simulink model "a1_climbing_new_swing"  (R2022b)
settings: Solver=ode15s  StartTime=0.0  StopTime=10  RelTol=1e-3
values from neighbouring files (symbols this model uses):
  m = 12    [MPC_Controller.m]    (also in QP_Controller.m; TASK1_rotating_mpc.m; TASK1_walking_backward_mpc.m; TASK1_walking_forward_mpc.m)
  N = 10    [MPC_Controller.m]
undefined symbols (not defined in the file or in its folder): climbing_mpc, square_trajectory_t_end, X, Y, Z
libraries: sm_lib x207, nesl_utility x134, simulink x1
(part 6 of 6)

== system a1_climbing_new_swing/Stand Controller/Subsystem9 ==
  angle : Inport
  velocity : Inport  Port=2
  Add : Sum
  Constant1 : Constant  Value=-0.5
  Constant2 : Constant  Value=-5
  Constant3 : Constant  Value=0
  Product : Product
  Product1 : Product
  Saturation : Saturate  UpperLimit=33.5  LowerLimit=-33.5
  Subtract : Sum  Inputs=+-
  Torque : Outport
  wires:
  angle/1 -> Subtract/1
  Constant2/1 -> Product/2
  Subtract/1 -> Product/1
  Constant1/1 -> Product1/2
  velocity/1 -> Product1/1
  Product1/1 -> Add/2
  Product/1 -> Add/1
  Constant3/1 -> Subtract/2
  Add/1 -> Saturation/1
  Saturation/1 -> Torque/1

== system a1_climbing_new_swing/Walk Controller/Convert Forces to Torque1 ==
  F : Inport
  RR_Ang_Vec : Inport  Port=2
  RL_Ang_Vec : Inport  Port=3
  FL_Ang_Vec : Inport  Port=4
  FR_Ang_Vec : Inport  Port=5
  Force to Torque : MATLAB Function  TreatAsAtomicUnit=on
  Tau_FL : Outport
  Tau_RL : Outport  Port=2
  Tau_FR : Outport  Port=3
  Tau_RR : Outport  Port=4
  wires:
  F/1 -> Force to Torque/1(F)
  Force to Torque/1(Tau_RR) -> Tau_RR/1
  Force to Torque/2(Tau_FR) -> Tau_FR/1
  Force to Torque/3(Tau_FL) -> Tau_FL/1
  Force to Torque/4(Tau_RL) -> Tau_RL/1
  RR_Ang_Vec/1 -> Force to Torque/2(RR_ang_vec)
  RL_Ang_Vec/1 -> Force to Torque/3(RL_ang_vec)
  FL_Ang_Vec/1 -> Force to Torque/4(FL_ang_vec)
  FR_Ang_Vec/1 -> Force to Torque/5(FR_ang_vec)

== system a1_climbing_new_swing/Walk Controller/Rigid Body Controller ==
  FL Pos : Inport
  RL Pos : Inport  Port=2
  FR Pos : Inport  Port=3
  RR Pos : Inport  Port=4
  COM_pos : Inport  Port=5
  COM_vel : Inport  Port=6
  COM_ang_vel : Inport  Port=7
  Rot : Inport  Port=8
  v_desired : Inport  Port=9
  T_stance : Inport  Port=10
  Clock : Clock
  Interpreted MATLAB Function : MATLABFcn  MATLABFcn=climbing_mpc(u)  OutputDimensions=12  Output1D=off
  Memory : Memory
  Mux : Mux  Inputs=11
  Rotation Matrix to Eul : MATLAB Function  TreatAsAtomicUnit=on
  Scope : Scope  NumInputPorts=5
  Selector : Selector  InputPortWidth=12  IndexOptions=Index vector (dialog)  Indices=[1 3]  OutputSizes=1
  Zero-Order Hold : ZeroOrderHold  SampleTime=.05
  u : Outport
  wires:
  COM_pos/1 -> Mux/1
  COM_vel/1 -> Mux/2
  COM_ang_vel/1 -> Mux/4
  FL Pos/1 -> Mux/5
  RL Pos/1 -> Mux/6
  FR Pos/1 -> Mux/7
  RR Pos/1 -> Mux/8
  Rot/1 -> Rotation Matrix to Eul/1(u)
  Rotation Matrix to Eul/1(y) -> Mux/3
  Interpreted MATLAB Function/1 -> Memory/1
  Memory/1 -> Selector/1, u/1
  Mux/1 -> Zero-Order Hold/1
  Zero-Order Hold/1 -> Interpreted MATLAB Function/1
  Clock/1 -> Mux/9
  Selector/1 -> Scope/1
  v_desired/1 -> Mux/10
  T_stance/1 -> Mux/11

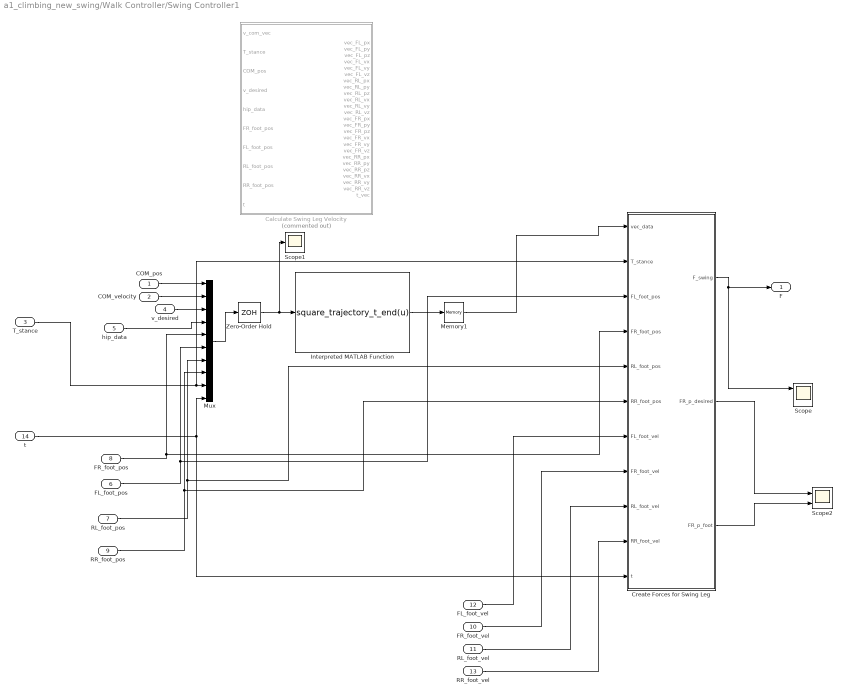
== system a1_climbing_new_swing/Walk Controller/Swing Controller1 ==
  COM_pos : Inport
  COM_velocity : Inport  Port=2
  T_stance : Inport  Port=3
  v_desired : Inport  Port=4
  hip_data : Inport  Port=5
  FL_foot_pos : Inport  Port=6
  RL_foot_pos : Inport  Port=7
  FR_foot_pos : Inport  Port=8
  RR_foot_pos : Inport  Port=9
  FR_foot_vel : Inport  Port=10
  RL_foot_vel : Inport  Port=11
  FL_foot_vel : Inport  Port=12
  RR_foot_vel : Inport  Port=13
  t : Inport  Port=14
  Calculate Swing Leg Velocity : MATLAB Function  Commented=on  TreatAsAtomicUnit=on
  Create Forces for Swing Leg : MATLAB Function  TreatAsAtomicUnit=on
  Interpreted MATLAB Function : MATLABFcn  MATLABFcn=square_trajectory_t_end(u)  OutputDimensions=1025  Output1D=off
  Memory1 : Memory
  Mux : Mux  Inputs=10
  Scope : Scope  NumInputPorts=3
  Scope1 : Scope
  Scope2 : Scope  NumInputPorts=2
  Zero-Order Hold : ZeroOrderHold  SampleTime=.2
  F : Outport
  wires:
  Create Forces for Swing Leg/1(F_swing) -> Scope/1, F/1
  t/1 -> Mux/10, Create Forces for Swing Leg/11(t)
  FR_foot_pos/1 -> Mux/5, Create Forces for Swing Leg/4(FR_foot_pos)
  RL_foot_pos/1 -> Mux/7, Create Forces for Swing Leg/5(RL_foot_pos)
  RR_foot_pos/1 -> Create Forces for Swing Leg/6(RR_foot_pos), Mux/8
  FL_foot_vel/1 -> Create Forces for Swing Leg/7(FL_foot_vel)
  FR_foot_vel/1 -> Create Forces for Swing Leg/8(FR_foot_vel)
  RL_foot_vel/1 -> Create Forces for Swing Leg/9(RL_foot_vel)
  RR_foot_vel/1 -> Create Forces for Swing Leg/10(RR_foot_vel)
  Create Forces for Swing Leg/2(FR_p_desired) -> Scope2/1
  Create Forces for Swing Leg/3(FR_p_foot) -> Scope2/2
  FL_foot_pos/1 -> Mux/6, Create Forces for Swing Leg/3(FL_foot_pos)
  Interpreted MATLAB Function/1 -> Memory1/1
  Zero-Order Hold/1 -> Scope1/1, Interpreted MATLAB Function/1
  COM_pos/1 -> Mux/1
  COM_velocity/1 -> Mux/2
  v_desired/1 -> Mux/3
  hip_data/1 -> Mux/4
  T_stance/1 -> Create Forces for Swing Leg/2(T_stance), Mux/9
  Mux/1 -> Zero-Order Hold/1
  Memory1/1 -> Create Forces for Swing Leg/1(vec_data)

== matlab function a1_climbing_new_swing/Rear Left Leg/Separate Torques ==
  data: torque_vector input; hip_torque output; thigh_torque output; calf_torque output
function [hip_torque, thigh_torque, calf_torque] = fcn(torque_vector)

hip_torque = torque_vector(1);
thigh_torque = torque_vector(2);
calf_torque = torque_vector(3);

== matlab function a1_climbing_new_swing/Front Right Leg/Separate Torques ==
  data: torque_vector input; hip_torque output; thigh_torque output; calf_torque output
function [hip_torque, thigh_torque, calf_torque] = fcn(torque_vector)

hip_torque = torque_vector(1);
thigh_torque = torque_vector(2);
calf_torque = torque_vector(3);

== matlab function a1_climbing_new_swing/Rear Right Leg/Separate Torques ==
  data: torque_vector input; hip_torque output; thigh_torque output; calf_torque output
function [hip_torque, thigh_torque, calf_torque] = fcn(torque_vector)

hip_torque = torque_vector(1);
thigh_torque = torque_vector(2);
calf_torque = torque_vector(3);

== matlab function a1_climbing_new_swing/Front Left Leg/Separate Torques ==
  data: torque_vector input; hip_torque output; thigh_torque output; calf_torque output
function [hip_torque, thigh_torque, calf_torque] = fcn(torque_vector)

hip_torque = torque_vector(1);
thigh_torque = torque_vector(2);
calf_torque = torque_vector(3);

== matlab function a1_climbing_new_swing/Stand Controller/MATLAB Function ==
  data: angle_vector input; hip_angle output; thigh_angle output; calf_angle output
function [hip_angle, thigh_angle, calf_angle] = fcn(angle_vector)

hip_angle = angle_vector(1);
thigh_angle = angle_vector(2);
calf_angle = angle_vector(3);

== matlab function a1_climbing_new_swing/Stand Controller/MATLAB Function1 ==
  data: velocity_vector input; hip_velocity output; thigh_velocity output; calf_velocity output
function [hip_velocity, thigh_velocity, calf_velocity] = fcn(velocity_vector)

hip_velocity = velocity_vector(1);
thigh_velocity = velocity_vector(2);
calf_velocity = velocity_vector(3);

== matlab function a1_climbing_new_swing/Stand Controller/MATLAB Function2 ==
  data: angle_vector input; hip_angle output; thigh_angle output; calf_angle output
function [hip_angle, thigh_angle, calf_angle] = fcn(angle_vector)

hip_angle = angle_vector(1);
thigh_angle = angle_vector(2);
calf_angle = angle_vector(3);

== matlab function a1_climbing_new_swing/Stand Controller/MATLAB Function3 ==
  data: velocity_vector input; hip_velocity output; thigh_velocity output; calf_velocity output
function [hip_velocity, thigh_velocity, calf_velocity] = fcn(velocity_vector)

hip_velocity = velocity_vector(1);
thigh_velocity = velocity_vector(2);
calf_velocity = velocity_vector(3);

== matlab function a1_climbing_new_swing/Stand Controller/MATLAB Function4 ==
  data: angle_vector input; hip_angle output; thigh_angle output; calf_angle output
function [hip_angle, thigh_angle, calf_angle] = fcn(angle_vector)

hip_angle = angle_vector(1);
thigh_angle = angle_vector(2);
calf_angle = angle_vector(3);

== matlab function a1_climbing_new_swing/Stand Controller/MATLAB Function5 ==
  data: velocity_vector input; hip_velocity output; thigh_velocity output; calf_velocity output
function [hip_velocity, thigh_velocity, calf_velocity] = fcn(velocity_vector)

hip_velocity = velocity_vector(1);
thigh_velocity = velocity_vector(2);
calf_velocity = velocity_vector(3);

== matlab function a1_climbing_new_swing/Stand Controller/MATLAB Function6 ==
  data: angle_vector input; hip_angle output; thigh_angle output; calf_angle output
function [hip_angle, thigh_angle, calf_angle] = fcn(angle_vector)

hip_angle = angle_vector(1);
thigh_angle = angle_vector(2);
calf_angle = angle_vector(3);

== matlab function a1_climbing_new_swing/Stand Controller/MATLAB Function7 ==
  data: velocity_vector input; hip_velocity output; thigh_velocity output; calf_velocity output
function [hip_velocity, thigh_velocity, calf_velocity] = fcn(velocity_vector)

hip_velocity = velocity_vector(1);
thigh_velocity = velocity_vector(2);
calf_velocity = velocity_vector(3);

== matlab function a1_climbing_new_swing/Walk Controller/Combine Forces ==
  data: t input; T_stance input; F output; rigid_body_forces input; swing_forces input; Contact input; Stair_Cont input
function F = fcn(t, T_stance, rigid_body_forces, swing_forces, Contact, Stair_Cont)
%#codegen
intervals = 0:T_stance:10;

interval_idx = discretize(t, intervals);
Stair1_Cont = Stair_Cont(1:4); Stair2_Cont = Stair_Cont(5:8); 


if Contact(1) == 0 && Stair1_Cont(1) == 0 && Stair2_Cont(1) == 0
    rigid_body_forces(1) = 0; 
end
if Contact(2) == 0 && Stair1_Cont(2) == 0 && Stair2_Cont(2) == 0 
    rigid_body_forces(4) = 0; 
end
if Contact(3) == 0 && Stair1_Cont(3) == 0 && Stair2_Cont(3) == 0 
    rigid_body_forces(7) = 0; 
end
if Contact(4) == 0 && Stair1_Cont(4) == 0 && Stair2_Cont(4) == 0 
    rigid_body_forces(10) = 0; 
end

if mod(interval_idx(1), 2) == 0
    F = [rigid_body_forces(1:3); -swing_forces(4:6); -swing_forces(7:9); rigid_body_forces(10:12)];
else
    F = [-swing_forces(1:3); rigid_body_forces(4:6); rigid_body_forces(7:9); -swing_forces(10:12)];
end

== matlab function a1_climbing_new_swing/Walk Controller/Rigid Body Controller/Rotation Matrix to Eul ==
  data: u input; y output
function y = fcn(u)
y = rotm2eul(u);

== matlab function a1_climbing_new_swing/Walk Controller/Swing Controller1/Calculate Swing Leg Velocity ==
  settings: updateMethod=CONTINUOUS
  data: vec_FL_px output size=41; vec_FL_py output size=41 [1..1000]; v_com_vec input; vec_FL_pz output size=41 [1..1000]; T_stance input; COM_pos input; v_desired input; hip_data input; FR_foot_pos input; FL_foot_pos input; RL_foot_pos input; vec_FL_vx output size=41; vec_FL_vy output size=41; vec_FL_vz output size=41; vec_RL_px output size=41; vec_RL_py output size=41; vec_RL_pz output size=41; vec_RL_vx output size=41; vec_RL_vy output size=41; vec_RL_vz output size=41; vec_FR_px output size=41; vec_FR_py output size=41; vec_FR_pz output size=41; vec_FR_vx output size=41; vec_FR_vy output size=41; vec_FR_vz output size=41; vec_RR_px output size=41; vec_RR_py output size=41; vec_RR_pz output size=41; vec_RR_vx output size=41; vec_RR_vy output size=41; vec_RR_vz output size=41; t_vec output size=41; RR_foot_pos input; t input
function [vec_FL_px,vec_FL_py,vec_FL_pz,vec_FL_vx,vec_FL_vy,vec_FL_vz,vec_RL_px,vec_RL_py,vec_RL_pz,vec_RL_vx,vec_RL_vy,vec_RL_vz,vec_FR_px,vec_FR_py,vec_FR_pz,vec_FR_vx,vec_FR_vy,vec_FR_vz,vec_RR_px,vec_RR_py,vec_RR_pz,vec_RR_vx,vec_RR_vy,vec_RR_vz,t_vec] = fcn(v_com_vec,T_stance,COM_pos,v_desired,hip_data,FR_foot_pos,FL_foot_pos,RL_foot_pos,RR_foot_pos,t)

z_height = 0.12; 

FL_hip_pos = hip_data(1:3);
FR_hip_pos = hip_data(4:6);
RL_hip_pos = hip_data(7:9);
RR_hip_pos = hip_data(10:12);
y_offset = 0.09; 

% Find K_step - this value can be tuned with z_com_desired
z_com_desired = 0.3;
t_delta = 0.005; 
g = 9.81;
K_step = sqrt(z_com_desired/g);

%% FL
% Find P_foot_desired - FL
FL_hip_pos(3) = 0;
FL_p_foot_desired_end = FL_hip_pos+(T_stance/2)*v_desired+K_step*(v_com_vec-v_desired);
FL_p_foot_desired_end(2) = FL_p_foot_desired_end(2)+y_offset;

if FL_p_foot_desired_end(1) > 0.4
    FL_p_foot_desired_end(3) = 0.1;
    half_step = (FL_p_foot_desired_end - FL_foot_pos)/2+[0;0;z_height];
elseif FL_p_foot_desired_end(1) > 0.6
    FL_p_foot_desired_end(3) = 0.2;
    half_step = (FL_p_foot_desired_end - FL_foot_pos)/2+[0;0;z_height];
else
   FL_p_foot_desired_end(3) = 0;
   half_step = (FL_p_foot_desired_end - FL_foot_pos)/2+[0;0;z_height];
end

% Create Velocity  
half_step_time = T_stance/2;
v = half_step/half_step_time;

% Create Trajectory Vectors
i = 1; 
vec_leng = 0:t_delta:T_stance;

vec_FL_px = zeros(1,length(vec_leng));
vec_FL_py = zeros(1,length(vec_leng));
vec_FL_pz = zeros(1,length(vec_leng));
vec_FL_vx = zeros(1,length(vec_leng));
vec_FL_vy = zeros(1,length(vec_leng));
vec_FL_vz = zeros(1,length(vec_leng));
t_vec = zeros(1,length(vec_leng));

for t = 0:t_delta:T_stance
    vec_FL_px(i) = v(1)*t;
    vec_FL_py(i) = v(2)*t;
    vec_FL_pz(i) = v(3)*t;
    vec_FL_vx(i) = v(1);
    vec_FL_vy(i) = v(2);
    vec_FL_vz(i) = v(3);
    t_vec(i) = t;
    if vec_FL_pz(i) > z_height
        vec_FL_pz(i) = z_height-v(3)*(t-T_stance/2);
        vec_FL_vz(i) = -v(3);
    end
    i = i+1; 
end

%% FR
% Find P_foot_desired - FR
FR_hip_pos(3) = 0;
FR_p_foot_desired_end = FR_hip_pos+(T_stance/2)*v_desired+K_step*(v_com_vec-v_desired);
FR_p_foot_desired_end(2) = FR_p_foot_desired_end(2)-y_offset;

if FR_p_foot_desired_end(1) > 0.4
    FR_p_foot_desired_end(3) = 0.1;
    half_step = (FR_p_foot_desired_end - FR_foot_pos)/2+[0;0;z_height];
elseif FR_p_foot_desired_end(1) > 0.6
    FR_p_foot_desired_end(3) = 0.2;
    half_step = (FR_p_foot_desired_end - FR_foot_pos)/2+[0;0;z_height];
else
   FR_p_foot_desired_end(3) = 0;
   half_step = (FR_p_foot_desired_end - FR_foot_pos)/2+[0;0;z_height];
end


% Create Trajectory 
half_step_time = T_stance/2;
v = half_step/half_step_time;


vec_FR_px = zeros(1,length(vec_leng));
vec_FR_py = zeros(1,length(vec_leng));
vec_FR_pz = zeros(1,length(vec_leng));
vec_FR_vx = zeros(1,length(vec_leng));
vec_FR_vy = zeros(1,length(vec_leng));
vec_FR_vz = zeros(1,length(vec_leng));

i = 1; 
for t = 0:t_delta:T_stance
    vec_FR_px(i) = v(1)*t;
    vec_FR_py(i) = v(2)*t;
    vec_FR_pz(i) = v(3)*t;
    vec_FR_vx(i) = v(1);
    vec_FR_vy(i) = v(2);
    vec_FR_vz(i) = v(3);
    if vec_FR_pz(i) > z_height
        vec_FR_pz(i) = z_height-v(3)*(t-T_stance/2);
        vec_FR_vz(i) = -v(3);
    end
    i = i+1; 
end

%% RL
% Find P_foot_desired - RL
RL_hip_pos(3) = 0;
RL_p_foot_desired_end = RL_hip_pos+(T_stance/2)*v_desired+K_step*(v_com_vec-v_desired);
RL_p_foot_desired_end(2) = RL_p_foot_desired_end(2)+y_offset;

if RL_p_foot_desired_end(1) > 0.4
    RL_p_foot_desired_end(3) = 0.1;
    half_step = (RL_p_foot_desired_end - RL_foot_pos)/2+[0;0;z_height];
elseif RL_p_foot_desired_end(1) > 0.6
    RL_p_foot_desired_end(3) = 0.2;
    half_step = (RL_p_foot_desired_end - RL_foot_pos)/2+[0;0;z_height];
else
   RL_p_foot_desired_end(3) = 0;
   half_step = (RL_p_foot_desired_end - RL_foot_pos)/2+[0;0;z_height];
end

% Create Trajectory 
half_step_time = T_stance/2;
v = half_step/half_step_time;


vec_RL_px = zeros(1,length(vec_leng));
vec_RL_py = zeros(1,length(vec_leng));
vec_RL_pz = zeros(1,length(vec_leng));
vec_RL_vx = zeros(1,length(vec_leng));
vec_RL_vy = zeros(1,length(vec_leng));
vec_RL_vz = zeros(1,length(vec_leng));
i = 1; 
for t = 0:t_delta:T_stance
    vec_RL_px(i) = v(1)*t;
    vec_RL_py(i) = v(2)*t;
    vec_RL_pz(i) = v(3)*t;
    vec_RL_vx(i) = v(1);
    vec_RL_vy(i) = v(2);
    vec_RL_vz(i) = v(3);
    if vec_RL_pz(i) > z_height
        vec_RL_pz(i) = z_height-v(3)*(t-T_stance/2);
        vec_RL_vz(i) = -v(3);
    end
    i = i+1; 
end


%% RR
% Find P_foot_desired - RR
RR_hip_pos(3) = 0;
RR_p_foot_desired_end = RR_hip_pos+(T_stance/2)*v_desired+K_step*(v_com_vec-v_desired);
RR_p_foot_desired_end(2) = RR_p_foot_desired_end(2)-y_offset;

% Create Trajectory 
if RR_p_foot_desired_end(1) > 0.4
    RR_p_foot_desired_end(3) = 0.1;
    half_step = (RR_p_foot_desired_end - RR_foot_pos)/2+[0;0;z_height];
elseif RR_p_foot_desired_end(1) > 0.6
    RR_p_foot_desired_end(3) = 0.2;
    half_step = (RR_p_foot_desired_end - RR_foot_pos)/2+[0;0;z_height];
else
   RR_p_foot_desired_end(3) = 0;
   half_step = (RR_p_foot_desired_end - RR_foot_pos)/2+[0;0;z_height];
end

half_step_time = T_stance/2;
v = half_step/half_step_time;


vec_RR_px = zeros(1,length(vec_leng));
vec_RR_py = zeros(1,length(vec_leng));
vec_RR_pz = zeros(1,length(vec_leng));
vec_RR_vx = zeros(1,length(vec_leng));
vec_RR_vy = zeros(1,length(vec_leng));
vec_RR_vz = zeros(1,length(vec_leng));
i = 1; 
for t = 0:t_delta:T_stance
    vec_RR_px(i) = v(1)*t;
    vec_RR_py(i) = v(2)*t;
    vec_RR_pz(i) = v(3)*t;
    vec_RR_vx(i) = v(1);
    vec_RR_vy(i) = v(2);
    vec_RR_vz(i) = v(3);
    if vec_FR_pz(i) > z_height
        vec_RR_pz(i) = z_height-v(3)*(t-T_stance/2);
        vec_RR_vz(i) = -v(3);
    end
    i = i+1; 
end

== matlab function a1_climbing_new_swing/Walk Controller/Swing Controller1/Create Forces for Swing Leg ==
  data: vec_data input size=[1025 1] [1..1000]; F_swing output; T_stance input; FL_foot_pos input; FR_foot_pos input; RL_foot_pos input; RR_foot_pos input; FL_foot_vel input; FR_foot_vel input; RL_foot_vel input; RR_foot_vel input; t input; FR_p_desired output; FR_p_foot output
function [F_swing,FR_p_desired,FR_p_foot]  = fcn(vec_data,T_stance,FL_foot_pos,FR_foot_pos,RL_foot_pos,RR_foot_pos,FL_foot_vel,FR_foot_vel,RL_foot_vel,RR_foot_vel,t)

% These are the desired velocity values calculated from the previous block
% These are the desired velocity for each foot position through the swing
vec_FL = vec_data(1:246);
vec_FL_px = vec_FL(1:41);
vec_FL_py = vec_FL(42:82);
vec_FL_pz = vec_FL(83:123);
vec_FL_vx = vec_FL(124:164);
vec_FL_vy = vec_FL(165:205);
vec_FL_vz = vec_FL(206:246);

vec_RL = vec_data(247:492);
vec_RL_px = vec_RL(1:41);
vec_RL_py = vec_RL(42:82);
vec_RL_pz = vec_RL(83:123);
vec_RL_vx = vec_RL(124:164);
vec_RL_vy = vec_RL(165:205);
vec_RL_vz = vec_RL(206:246);

vec_FR = vec_data(493:738);
vec_FR_px = vec_FR(1:41);
vec_FR_py = vec_FR(42:82);
vec_FR_pz = vec_FR(83:123);
vec_FR_vx = vec_FR(124:164);
vec_FR_vy = vec_FR(165:205);
vec_FR_vz = vec_FR(206:246);

vec_RR = vec_data(739:984);
vec_RR_px = vec_RR(1:41);
vec_RR_py = vec_RR(42:82);
vec_RR_pz = vec_RR(83:123);
vec_RR_vx = vec_RR(124:164);
vec_RR_vy = vec_RR(165:205);
vec_RR_vz = vec_RR(206:246);

t_vec = vec_data(985:1025);


steps = 0:T_stance:10;
step_index = discretize(t,steps);
delta_t = t-steps(step_index);

[dt index] = min(abs(t_vec-delta_t));


FL_v_desired = [vec_FL_vx(index);vec_FL_vy(index);vec_FL_vz(index)];
FR_v_desired = [vec_FR_vx(index);vec_FR_vy(index);vec_FR_vz(index)];
RL_v_desired = [vec_RL_vx(index);vec_RL_vy(index);vec_RL_vz(index)];
RR_v_desired = [vec_RR_vx(index);vec_RR_vy(index);vec_RR_vz(index)];

FL_p_desired = [vec_FL_px(index);vec_FL_py(index);vec_FL_pz(index)];
FR_p_desired = [vec_FR_px(index);vec_FR_py(index);vec_FR_pz(index)];
RL_p_desired = [vec_RL_px(index);vec_RL_py(index);vec_RL_pz(index)];
RR_p_desired = [vec_RR_px(index);vec_RR_py(index);vec_RR_pz(index)];


% These are the actual current foot position and velocity - these update
% continously
FL_p_foot = FL_foot_pos(1:3);
FL_v_foot = FL_foot_vel(1:3);
FR_p_foot = FR_foot_pos(1:3);
FR_v_foot = FR_foot_vel(1:3);
RL_p_foot = RL_foot_pos(1:3);
RL_v_foot = RL_foot_vel(1:3);
RR_p_foot = RR_foot_pos(1:3);
RR_v_foot = RR_foot_vel(1:3);

% Find the force using a PD controller - FL
KP = [1300;400;2000]; 
KD = [12;10;20]; 
F_swing_FL = KP.*(FL_p_desired-FL_p_foot)+KD.*(FL_v_desired-FL_v_foot);
F_swing_FR = KP.*(FR_p_desired-FR_p_foot)+KD.*(FR_v_desired-FR_v_foot);
F_swing_RL = KP.*(RL_p_desired-RL_p_foot)+KD.*(RL_v_desired-RL_v_foot);
F_swing_RR = KP.*(RR_p_desired-RR_p_foot)+KD.*(RR_v_desired-RR_v_foot);

F_swing = [F_swing_FL;F_swing_RL; F_swing_FR; F_swing_RR];

== matlab function a1_climbing_new_swing/Walk Controller/MATLAB Function ==
  data: P input; pos_d output; v_d input
function pos_d = fcn(P,v_d)
dt = 0.05;
pos_d = P(1)+ 10*dt*v_d(1);

== matlab function a1_climbing_new_swing/MATLAB Function ==
  data: t input; FL output; torques_stand input; torques_walk input; RL output; FR output; RR output
function [FL, RL, FR, RR] = fcn(t, torques_stand, torques_walk)
%#codegen
if t < 1
    FL = torques_stand(1:3);
    RL = torques_stand(4:6);
    FR = torques_stand(7:9);
    RR = torques_stand(10:12);
else
    FL = torques_walk(1:3);
    RL = torques_walk(4:6);
    FR = torques_walk(7:9);
    RR = torques_walk(10:12);
end

== matlab function a1_climbing_new_swing/Walk Controller/Convert Forces to Torque1/Force to Torque ==
  data: F input; Tau_RR output; RR_ang_vec input; RL_ang_vec input; FL_ang_vec input; FR_ang_vec input; Tau_FR output; Tau_FL output; Tau_RL output
function [Tau_RR,Tau_FR,Tau_FL,Tau_RL]= fcn(F,RR_ang_vec,RL_ang_vec,FL_ang_vec,FR_ang_vec)
    % TODO - Convert forces to torques using the inverse jacobian
    % Get forces from the force vector 
    % NOTE - VERIFY THAT THESE ARE THE CORRECT VECTORS (I am unsure)
    F_FL = F(1:3);
    F_RL = F(4:6);
    F_FR = F(7:9);
    F_RR = F(10:12);

    l1=0.045; % hip length
    l2=0.2; % thigh length
    l3=0.2; % calf length
    

    %% Calculate the force for the RR leg - NOTE: The right legs have the
    % same jacobians
    q = RR_ang_vec; %
    leg = 4;
  
    if leg==1 || leg==3 % left leg has sideSign 1
        sideSign=1;
    else
        sideSign=-1; % right leg has sideSign -1
    end
    s1=sin(q(1)); % for hip joint
    s2=sin(q(2)); % for thigh joint
    s3=sin(q(3)); % for calf joint

    c1=cos(q(1)); % for hip joint
    c2=cos(q(2)); % for thigh joint
    c3=cos(q(3)); % for calf joint
    
    c23=c2*c3-s2*s3;
    s23=s2*c3+c2*s3;
    J = eye(3);
    J(1,1)=0;
    J(2,1)=-sideSign*l1*s1+l2*c2*c1+l3*c23*c1;
    J(3,1)=sideSign*l1*c1+l2*c2*s1+l3*c23*s1;
    
    J(1,2)=-l3*c23-l2*c2;
    J(2,2)=-l2*s2*s1-l3*s23*s1;
    J(3,2)=l2*s2*c1+l3*s23*c1;

    J(1,3)=-l3*c23;
    J(2,3)=-l3*s23*s1;
    J(3,3)=l3*s23*c1;
    
    inJ_R_RR = transpose(J);
    Tau_RR = -inJ_R_RR*F_RR;

  
    %% Calculate the force for the FR leg - NOTE: The right legs have the
    % same jacobians
    q = FR_ang_vec; %
    leg = 2;
  
    if leg==1 || leg==3 % left leg has sideSign 1
        sideSign=1;
    else
        sideSign=-1; % right leg has sideSign -1
    end
    s1=sin(q(1)); % for hip joint
    s2=sin(q(2)); % for thigh joint
    s3=sin(q(3)); % for calf joint

    c1=cos(q(1)); % for hip joint
    c2=cos(q(2)); % for thigh joint
    c3=cos(q(3)); % for calf joint
    
    c23=c2*c3-s2*s3;
    s23=s2*c3+c2*s3;

    J(1,1)=0;
    J(2,1)=-sideSign*l1*s1+l2*c2*c1+l3*c23*c1;
    J(3,1)=sideSign*l1*c1+l2*c2*s1+l3*c23*s1;
    
    J(1,2)=-l3*c23-l2*c2;
    J(2,2)=-l2*s2*s1-l3*s23*s1;
    J(3,2)=l2*s2*c1+l3*s23*c1;

    J(1,3)=-l3*c23;
    J(2,3)=-l3*s23*s1;
    J(3,3)=l3*s23*c1;

    inJ_R_FR = transpose(J);
    Tau_FR = -inJ_R_FR*F_FR;

    %% Calculate the force for the FL leg - NOTE: The right legs have the
    % same jacobians
    q = FL_ang_vec; %
    leg = 1;
  
    if leg==1 || leg==3 % left leg has sideSign 1
        sideSign=1;
    else
        sideSign=-1; % right leg has sideSign -1
    end
    s1=sin(q(1)); % for hip joint
    s2=sin(q(2)); % for thigh joint
    s3=sin(q(3)); % for calf joint

    c1=cos(q(1)); % for hip joint
    c2=cos(q(2)); % for thigh joint
    c3=cos(q(3)); % for calf joint
    
    c23=c2*c3-s2*s3;
    s23=s2*c3+c2*s3;

    J(1,1)=0;
    J(2,1)=-sideSign*l1*s1+l2*c2*c1+l3*c23*c1;
    J(3,1)=sideSign*l1*c1+l2*c2*s1+l3*c23*s1;
    
    J(1,2)=-l3*c23-l2*c2;
    J(2,2)=-l2*s2*s1-l3*s23*s1;
    J(3,2)=l2*s2*c1+l3*s23*c1;

    J(1,3)=-l3*c23;
    J(2,3)=-l3*s23*s1;
    J(3,3)=l3*s23*c1;

    inJ_R_FL = transpose(J);
    Tau_FL = -inJ_R_FL*F_FL;


    %% Calculate the force for the RL leg - NOTE: The right legs have the
    % same jacobians
    q = RL_ang_vec; %
    leg = 3;
  
    if leg==1 || leg==3 % left leg has sideSign 1
        sideSign=1;
    else
        sideSign=-1; % right leg has sideSign -1
    end
    s1=sin(q(1)); % for hip joint
    s2=sin(q(2)); % for thigh joint
    s3=sin(q(3)); % for calf joint

    c1=cos(q(1)); % for hip joint
    c2=cos(q(2)); % for thigh joint
    c3=cos(q(3)); % for calf joint
    
    c23=c2*c3-s2*s3;
    s23=s2*c3+c2*s3;

    J(1,1)=0;
    J(2,1)=-sideSign*l1*s1+l2*c2*c1+l3*c23*c1;
    J(3,1)=sideSign*l1*c1+l2*c2*s1+l3*c23*s1;
    
    J(1,2)=-l3*c23-l2*c2;
    J(2,2)=-l2*s2*s1-l3*s23*s1;
    J(3,2)=l2*s2*c1+l3*s23*c1;

    J(1,3)=-l3*c23;
    J(2,3)=-l3*s23*s1;
    J(3,3)=l3*s23*c1;

    inJ_R_RL = transpose(J);
    Tau_RL = -inJ_R_RL*F_RL;
